simulink library "SelectorBlock"  (R2017a)
settings: Solver=VariableStepAuto  StartTime=0.0  StopTime=10.0  RelTol=1e-3
settings Model: Creator=hwinter  LastModifiedBy=hwinter

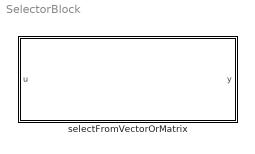
== system SelectorBlock ==
  selectFromVectorOrMatrix : Subsystem  mask{mv_row_selector=[1,2], mv_column_selector=1}
      mask prompts: mv_row_selector "Row selector:"; mv_column_selector "Column selector:"
      mask init:
      | mv_selector = [1:2,1];
      mask Display:
      | str1 = sprintf('\\color{black}{\\bfSelector Block}\n\n');
      | 
      | str2 = sprintf('Row selector: [');
      | str3 = sprintf(' %d',mv_row_selector);
      | str3 = sprintf('%s\n',[str3(2:end),']']);
      | 
      | str4 = sprintf('Column selector: [');
      | str5 = sprintf(' %d',mv_column_selector);
      | str5 = [str5(2:end),']'];
      | 
      | str = [str1,str2,str3,str4,str5];
      | 
      | text( 0.5,0.5, ...
      |       str, ...
      |       'horizontalAlignment', 'center', ...
      |       'texmode','on' ...
      |     )

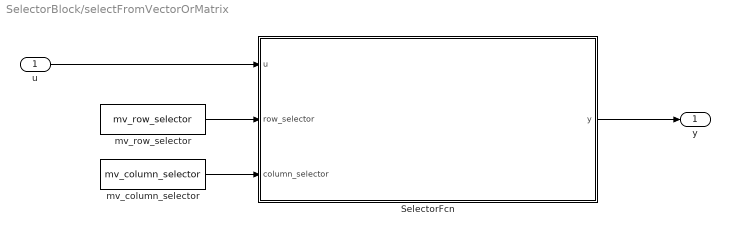
== system SelectorBlock/selectFromVectorOrMatrix ==
  u : Inport
  SelectorFcn : MATLAB Function  TreatAsAtomicUnit=on
  mv_column_selector : Constant  Value=mv_column_selector
  mv_row_selector : Constant  Value=mv_row_selector
  y : Outport
  wires:
  mv_column_selector/1 -> SelectorFcn/3(column_selector)
  SelectorFcn/1(y) -> y/1
  u/1 -> SelectorFcn/1(u)
  mv_row_selector/1 -> SelectorFcn/2(row_selector)

== matlab function SelectorBlock/selectFromVectorOrMatrix/SelectorFcn ==
  data: u input [1..1000]; y output size=[max_x_size max_x_size] [1..1000]; row_selector input; column_selector input; max_x_size parameter
function y = selectFromVectorOrMatrix(u,row_selector,column_selector,max_x_size)

coder.varsize('y',[max_x_size max_x_size]);

y = u(row_selector,column_selector);

end % end function selectFromVectorOrMatrix
